simulink model "variant_2_MRC_SimulationModel"  (R2015a)
settings: Solver=ode3  SolverMode=SingleTasking  StartTime=0.0  StopTime=180  RelTol=1e-3
PreLoadFcn:
  | addLibrariesInPath('sim')
PostLoadFcn:
  | loadRobotParameters
StartFcn:
  | simApp = SimDisplay.getInstance;
  | simApp.reset;
  | simApp.TrackView.setup(double(SitesPositions), ObstaclesPositions,ObstaclesVertices,ObstaclesEdges);
undefined symbols (not defined in the file): AngularSpeed, AxleLength, do_one_run, EncL_init, EncR_init, EncRes, lcam, motorDeadBand, motorL, motorR, motorX, ObstaclesEdges, ObstaclesVertices, pcam, SitesPositions, startPos, TauMotor, theta0, Ts, WheelRadius
libraries: simulink_extras x1, realtime_pacer_lib x1, simulink x1, cstblocks x1
(part 1 of 2)
CloseFcn:
  | delete(SimDisplay.getInstance());
settings Model: PauseTimes=14  CovSFcnEnable=off  ExtModeTrigDuration=2  Creator=gpacitti  LastModifiedBy=planger
settings OptimizationCC: BlockReduction=off  BooleanDataType=off
settings DebuggingCC: SaveWithParameterizedLinksMsg=none  SignalResolutionControl=TryResolveAllWithWarning  ParameterPrecisionLossMsg=none
settings HardwareCC: TargetUnknown=on

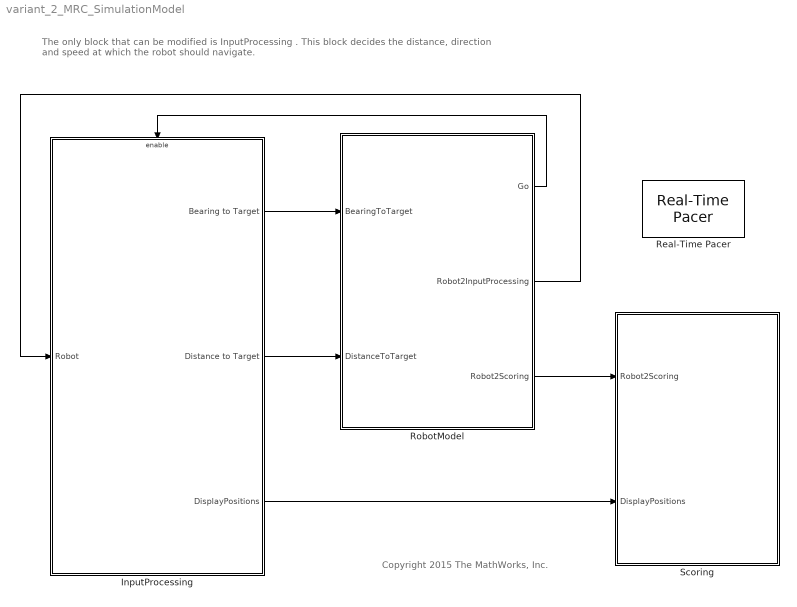
== system variant_2_MRC_SimulationModel ==
  note: Copyright 2015 The MathWorks, Inc.
  note: The only block that can be modified is InputProcessing .
      | This block decides the distance, direction and speed at which the robot should navigate.
  InputProcessing : Subsystem
      mask Display: image('Arduino_Due_2_0274.png',[0.15,0.3,0.45,0.4]);
  Real-Time Pacer : realtime_pacer_lib/Real-Time Pacer  simTimePerRealTime=1
  RobotModel : Subsystem  mask(Robot){}
      mask help:
      | !! DO NOT MODIFY !!
      | Model representing the robot behavior including physical representation and sensors.
      mask Display: image('robot_3d.jpg',[0.4,0.7,0.45,0.25]);
  Scoring : Subsystem  mask(Scoring){}
      mask help:
      | !! DO NOT MODIFY !!
      | Model representing the judge and visualisation.
  wires:
  InputProcessing/3(DisplayPositions) -> Scoring/2(DisplayPositions)
  InputProcessing/1(Bearing to Target) -> RobotModel/1(BearingToTarget)
  InputProcessing/2(Distance to Target) -> RobotModel/2(DistanceToTarget)
  RobotModel/2(Robot2InputProcessing) -> InputProcessing/1(Robot)
  RobotModel/3(Robot2Scoring) -> Scoring/1(Robot2Scoring)
  RobotModel/1(Go) -> InputProcessing/Enable

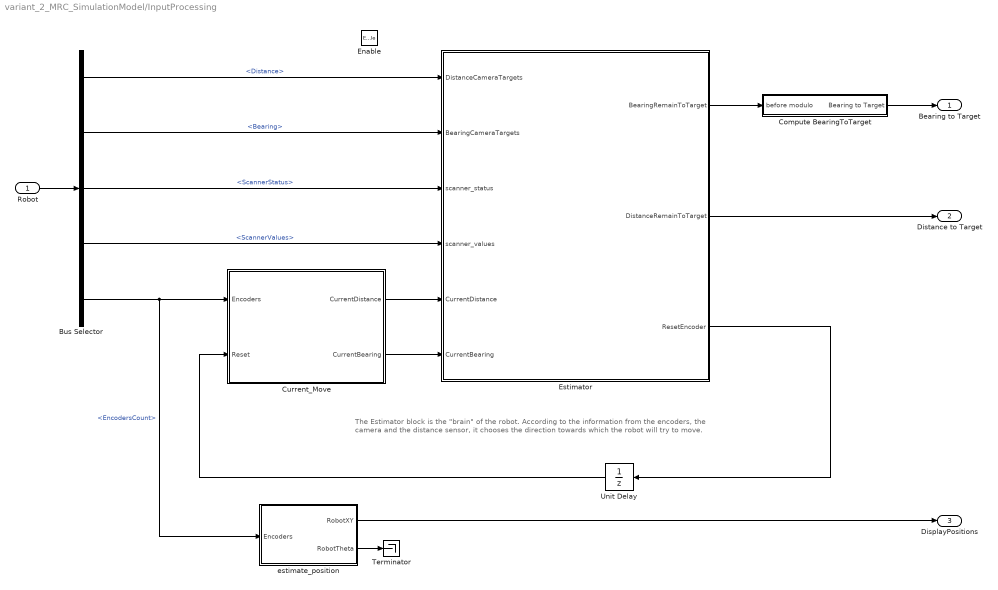
== system variant_2_MRC_SimulationModel/InputProcessing ==
  note: The Estimator block is the "brain" of the robot. According to the information from the encoders, the camera and the
      | distance sensor, it chooses the direction towards which the robot will try to move.
  Robot : Inport
  Enable : EnablePort  StatesWhenEnabling=reset
  Bus Selector : BusSelector  OutputSignals=Distance,Bearing,ScannerStatus,ScannerValues,EncodersCount
  Compute BearingToTarget : Subsystem
  Current_Move : Subsystem
  Estimator : Stateflow chart  TreatAsAtomicUnit=on
  Terminator : Terminator
  Unit Delay : UnitDelay  SampleTime=-1
  estimate_position : Subsystem
  Bearing to Target : Outport  SampleTime=Ts
  Distance to Target : Outport  Port=2
  DisplayPositions : Outport  Port=3
  wires:
  Robot/1 -> Bus Selector/1
  Bus Selector/1 -> Estimator/1(DistanceCameraTargets)  "<Distance>"
  Bus Selector/2 -> Estimator/2(BearingCameraTargets)  "<Bearing>"
  Estimator/1(BearingRemainToTarget) -> Compute BearingToTarget/1(before modulo)
  Estimator/2(DistanceRemainToTarget) -> Distance to Target/1
  Estimator/3(ResetEncoder) -> Unit Delay/1
  Unit Delay/1 -> Current_Move/2(Reset)
  Current_Move/1(CurrentDistance) -> Estimator/5(CurrentDistance)
  Compute BearingToTarget/1(Bearing to Target) -> Bearing to Target/1
  Current_Move/2(CurrentBearing) -> Estimator/6(CurrentBearing)
  estimate_position/2(RobotTheta) -> Terminator/1
  estimate_position/1(RobotXY) -> DisplayPositions/1
  Bus Selector/3 -> Estimator/3(scanner_status)  "<ScannerStatus>"
  Bus Selector/4 -> Estimator/4(scanner_values)  "<ScannerValues>"
  Bus Selector/5 -> estimate_position/1(Encoders), Current_Move/1(Encoders)  "<EncodersCount>"

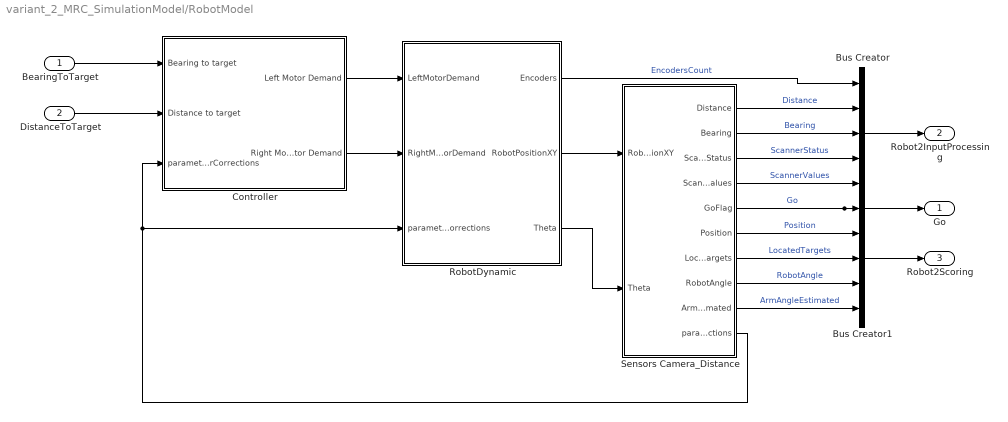
== system variant_2_MRC_SimulationModel/RobotModel ==
  BearingToTarget : Inport  SampleTime=0
  DistanceToTarget : Inport  Port=2  SampleTime=0
  Bus Creator : BusCreator  Inputs=5
  Bus Creator1 : BusCreator  Inputs=5
  Controller : Subsystem  TreatAsAtomicUnit=on
  RobotDynamic : Subsystem
  Sensors Camera_Distance : Subsystem
  Go : Outport
  Robot2InputProcessing : Outport  Port=2
  Robot2Scoring : Outport  Port=3
  wires:
  DistanceToTarget/1 -> Controller/2(Distance to target)
  BearingToTarget/1 -> Controller/1(Bearing to target)
  Bus Creator/1 -> Robot2InputProcessing/1
  Controller/1(Left Motor Demand) -> RobotDynamic/1(LeftMotorDemand)
  Controller/2(Right Motor Demand) -> RobotDynamic/2(RightMotorDemand)
  Bus Creator1/1 -> Robot2Scoring/1
  RobotDynamic/3(Theta) -> Sensors Camera_Distance/2(Theta)
  RobotDynamic/2(RobotPositionXY) -> Sensors Camera_Distance/1(RobotPositionXY)
  RobotDynamic/1(Encoders) -> Bus Creator/1  "EncodersCount"
  Sensors Camera_Distance/4(ScannerValues) -> Bus Creator/5  "ScannerValues"
  Sensors Camera_Distance/3(ScannerStatus) -> Bus Creator/4  "ScannerStatus"
  Sensors Camera_Distance/2(Bearing) -> Bus Creator/3  "Bearing"
  Sensors Camera_Distance/1(Distance) -> Bus Creator/2  "Distance"
  Sensors Camera_Distance/7(LocatedTargets) -> Bus Creator1/3  "LocatedTargets"
  Sensors Camera_Distance/8(RobotAngle) -> Bus Creator1/4  "RobotAngle"
  Sensors Camera_Distance/9(ArmAngleEstimated) -> Bus Creator1/5  "ArmAngleEstimated"
  Sensors Camera_Distance/10(parameterCorrections) -> RobotDynamic/3(parameterCorrections), Controller/3(parameterCorrections)
  Sensors Camera_Distance/6(Position) -> Bus Creator1/2  "Position"
  Sensors Camera_Distance/5(GoFlag) -> Bus Creator1/1, Go/1  "Go"

== system variant_2_MRC_SimulationModel/Scoring ==
  Robot2Scoring : Inport
  DisplayPositions : Inport  Port=2
  Bus Selector : BusSelector  OutputSignals=Position,Go
  Bus Selector1 : BusSelector  OutputSignals=LocatedTargets,RobotAngle,ArmAngleEstimated
  FigureOutput : Subsystem  TreatAsAtomicUnit=on  SimViewingDevice=on
  Referee : Subsystem
      mask Display: % image(imread('referee.png'))
  wires:
  Referee/1(Targets Located) -> FigureOutput/2(Targets Found)  "TargetsLocated"
  Referee/2(Time Last Target Found) -> FigureOutput/3(Time Last Found)  "TimeLastTargetFound"
  Referee/3(Elapsed Time_sec) -> FigureOutput/4(Time Elapsed)  "ElapsedTime"
  DisplayPositions/1 -> FigureOutput/9(DisplayPositions)
  Robot2Scoring/1 -> Bus Selector1/1, Bus Selector/1
  Bus Selector/2 -> Referee/2(Start Flag)  "<Go>"
  Bus Selector/1 -> FigureOutput/1(Position), Referee/1(Robot Position_m)  "<Position>"
  Bus Selector1/1 -> FigureOutput/5(locatedTargets)  "<LocatedTargets>"
  Bus Selector1/2 -> FigureOutput/6(robottheta)  "<RobotAngle>"
  Bus Selector1/3 -> FigureOutput/8(ArmAngleCommand), FigureOutput/7(ArmAngleEstimated)  "<ArmAngleEstimated>"

== system variant_2_MRC_SimulationModel/InputProcessing/Compute BearingToTarget ==
  before modulo : Inport
  Constant : Constant  Value=180  OutDataTypeStr=Inherit: Inherit via back propagation
  Constant1 : Constant  Value=360  OutDataTypeStr=Inherit: Inherit via back propagation
  Math Function1 : Math  Operator=mod  SaturateOnIntegerOverflow=on
  Sum10 : Sum  Inputs=-+|
  Sum7 : Sum  Inputs=++|
  Bearing to Target : Outport  SampleTime=Ts
  wires:
  Constant/1 -> Sum7/1, Sum10/1
  Sum7/1 -> Math Function1/1
  Constant1/1 -> Math Function1/2
  Math Function1/1 -> Sum10/2
  Sum10/1 -> Bearing to Target/1
  before modulo/1 -> Sum7/2

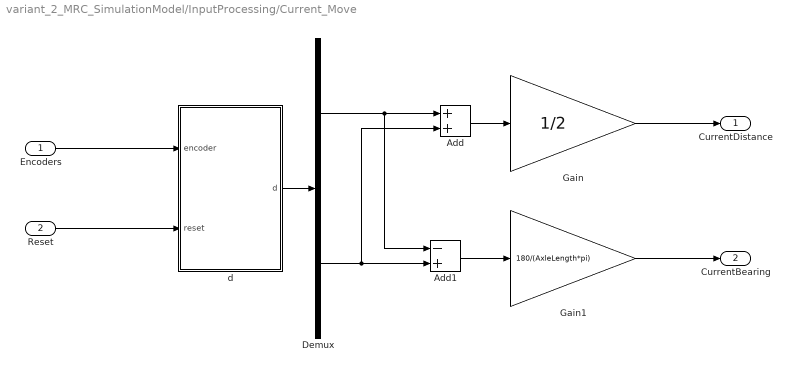
== system variant_2_MRC_SimulationModel/InputProcessing/Current_Move ==
  Encoders : Inport
  Reset : Inport  Port=2
  Add : Sum
  Add1 : Sum  Inputs=-+
  Demux : Demux  Outputs=2
  Gain : Gain  Gain=1/2
  Gain1 : Gain  Gain=180/(AxleLength*pi)
  d : Subsystem
  CurrentDistance : Outport
  CurrentBearing : Outport  Port=2
  wires:
  Reset/1 -> d/2(reset)
  Demux/2 -> Add/2, Add1/2
  Add1/1 -> Gain1/1
  Gain1/1 -> CurrentBearing/1
  Gain/1 -> CurrentDistance/1
  Demux/1 -> Add1/1, Add/1
  Add/1 -> Gain/1
  Encoders/1 -> d/1(encoder)
  d/1(d) -> Demux/1

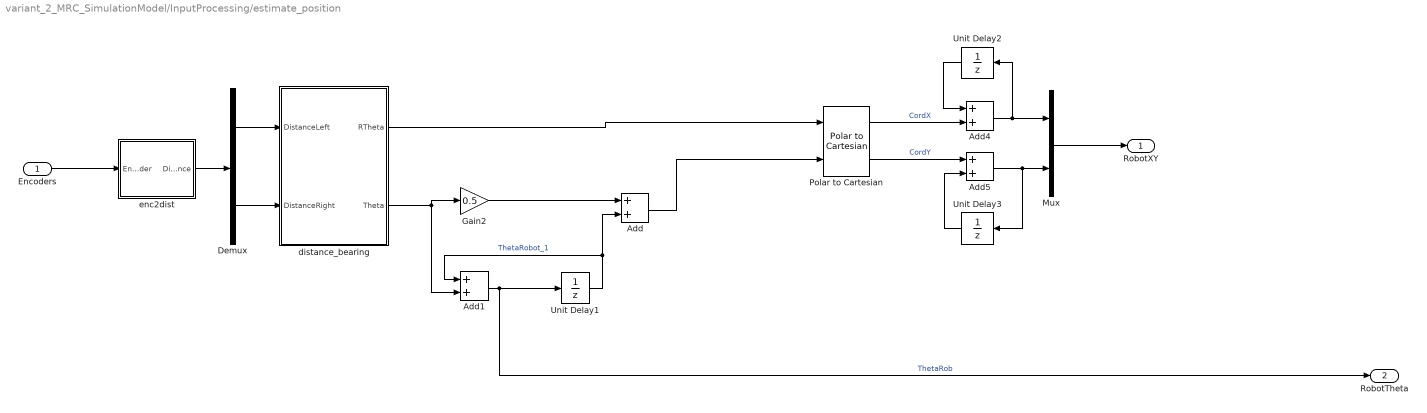
== system variant_2_MRC_SimulationModel/InputProcessing/estimate_position ==
  Encoders : Inport
  Add{,1,4..5} (4 alike) : Sum
  Demux : Demux  Outputs=2
  Gain2 : Gain  Gain=0.5
  Mux : Mux  Inputs=2
  Polar to Cartesian : simulink_extras/Transformations/Polar to Cartesian
  Unit Delay1 : UnitDelay  DialogController=Simulink.DDGSource  InitialCondition=theta0*pi/180  SampleTime=-1
  Unit Delay2 : UnitDelay  DialogController=Simulink.DDGSource  InitialCondition=single(startPos(1))  SampleTime=-1
  Unit Delay3 : UnitDelay  DialogController=Simulink.DDGSource  InitialCondition=single(startPos(2))  SampleTime=-1
  distance_bearing : Subsystem
  enc2dist : Subsystem
  RobotXY : Outport
  RobotTheta : Outport  Port=2
  wires:
  Gain2/1 -> Add/1
  Polar to Cartesian/1 -> Add4/2  "CordX"
  Polar to Cartesian/2 -> Add5/1  "CordY"
  Add4/1 -> Unit Delay2/1, Mux/1
  Unit Delay2/1 -> Add4/1
  Add5/1 -> Mux/2, Unit Delay3/1
  Unit Delay3/1 -> Add5/2
  distance_bearing/2(Theta) -> Gain2/1, Add1/2
  Unit Delay1/1 -> Add1/1, Add/2  "ThetaRobot_1"
  Add/1 -> Polar to Cartesian/2
  Add1/1 -> RobotTheta/1, Unit Delay1/1  "ThetaRob"
  distance_bearing/1(RTheta) -> Polar to Cartesian/1
  Mux/1 -> RobotXY/1
  enc2dist/1(Distance) -> Demux/1
  Demux/1 -> distance_bearing/1(DistanceLeft)
  Demux/2 -> distance_bearing/2(DistanceRight)
  Encoders/1 -> enc2dist/1(Encoder)

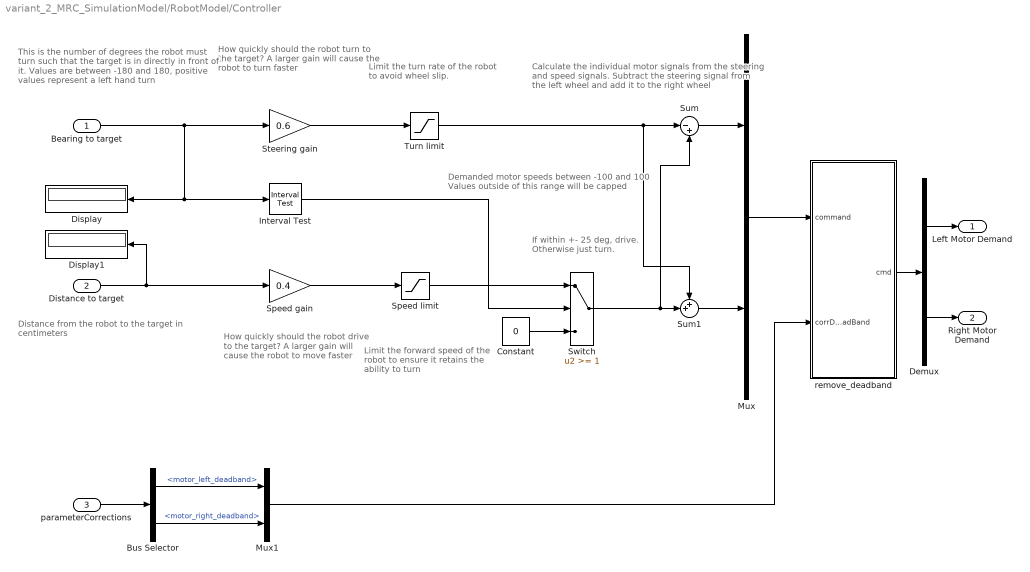
== system variant_2_MRC_SimulationModel/RobotModel/Controller ==
  note: Limit the turn rate of the
      | robot to avoid wheel slip.
  note: If within +- 25 deg, drive.
      | Otherwise just turn.
  note: Calculate the individual motor signals from the
      | steering and speed signals. Subtract the steering
      | signal from the left wheel and add it to the right
      | wheel
  note: Limit the forward speed of the
      | robot to ensure it retains the
      | ability to turn
  note: How quickly should the robot
      | drive to the target? A larger gain
      | will cause the robot to move
      | faster
  note: How quickly should the robot turn
      | to the target? A larger gain will
      |  cause the robot to turn faster
  note: Demanded motor speeds between -100 and 100
      | Values outside of this range will be capped
  note: Distance from the robot to the target
      | in centimeters
  note: This is the number of degrees the robot
      | must turn such that the target is in directly
      | in front of it.
      | Values are between -180 and 180,
      | positive values represent a left hand turn
  Bearing to target : Inport  OutDataTypeStr=single
  Distance to target : Inport  Port=2  PortDimensions=1  SampleTime=Ts
  parameterCorrections : Inport  Port=3  SampleTime=Ts
  Bus Selector : BusSelector  OutputSignals=motor_left_deadband,motor_right_deadband
  Constant : Constant  Value=0  OutDataTypeStr=single
  Demux : Demux  Outputs=2
  Display : Display
  Display1 : Display
  Interval Test : simulink/Logic and Bit Operations/Interval Test  IntervalClosedRight=on  uplimit=25  IntervalClosedLeft=on  lowlimit=-25  OutDataTypeStr=boolean
      settings: AttributesFormatString=|
      | Upper = %<uplimit>
      | Lower = %<lowlimit>
  Mux : Mux  Inputs=2
  Mux1 : Mux  Inputs=2
  Speed gain : Gain  Gain=0.4
  Speed limit : Saturate  UpperLimit=40  LowerLimit=0
      settings: AttributesFormatString=|
      | Upper = %<UpperLimit>
      | Lower = %<LowerLimit>
  Steering gain : Gain  Gain=0.6
  Sum : Sum  Inputs=|-+
  Sum1 : Sum  Inputs=++|
  Switch : Switch  Threshold=1
  Turn limit : Saturate  UpperLimit=50  LowerLimit=-50
      settings: AttributesFormatString=|
      | Upper = %<UpperLimit>
      | Lower = %<LowerLimit>
  remove_deadband : Subsystem
  Left Motor Demand : Outport  OutDataTypeStr=single
  Right Motor Demand : Outport  Port=2  OutDataTypeStr=single
  wires:
  Bearing to target/1 -> Steering gain/1, Display/1, Interval Test/1
  Speed gain/1 -> Speed limit/1
  Distance to target/1 -> Display1/1, Speed gain/1
  Steering gain/1 -> Turn limit/1
  Switch/1 -> Sum/2, Sum1/2
  Interval Test/1 -> Switch/2
  Constant/1 -> Switch/3
  Turn limit/1 -> Sum/1, Sum1/1
  Speed limit/1 -> Switch/1
  parameterCorrections/1 -> Bus Selector/1
  Sum1/1 -> Mux/2
  Sum/1 -> Mux/1
  Mux/1 -> remove_deadband/1(command)
  remove_deadband/1(cmd) -> Demux/1
  Demux/1 -> Left Motor Demand/1
  Demux/2 -> Right Motor Demand/1
  Bus Selector/1 -> Mux1/1  "<motor_left_deadband>"
  Bus Selector/2 -> Mux1/2  "<motor_right_deadband>"
  Mux1/1 -> remove_deadband/2(corrDeadBand)

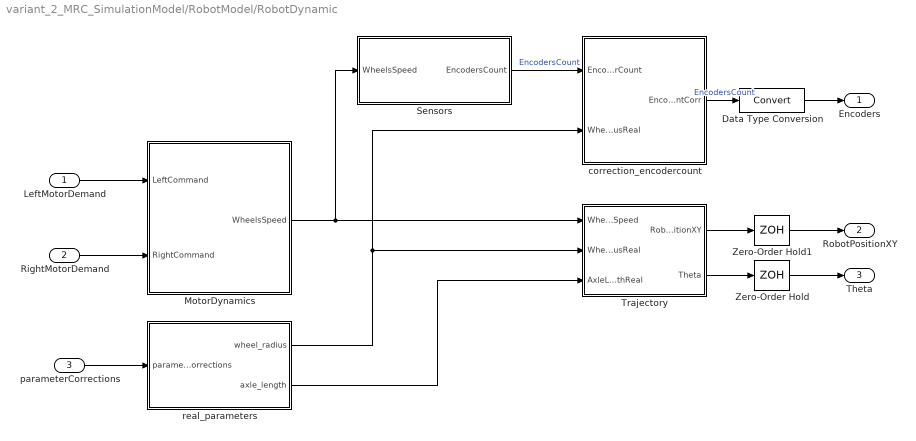
== system variant_2_MRC_SimulationModel/RobotModel/RobotDynamic ==
  LeftMotorDemand : Inport
  RightMotorDemand : Inport  Port=2
  parameterCorrections : Inport  Port=3
  Data Type Conversion : DataTypeConversion
  MotorDynamics : Subsystem
  Sensors : Subsystem
  Trajectory : Subsystem
  Zero-Order Hold : ZeroOrderHold  SampleTime=Ts
  Zero-Order Hold1 : ZeroOrderHold  SampleTime=Ts
  correction_encodercount : Subsystem
  real_parameters : Subsystem
  Encoders : Outport
  RobotPositionXY : Outport  Port=2
  Theta : Outport  Port=3
  wires:
  MotorDynamics/1(WheelsSpeed) -> Trajectory/1(WheelsSpeed), Sensors/1(WheelsSpeed)
  RightMotorDemand/1 -> MotorDynamics/2(RightCommand)
  LeftMotorDemand/1 -> MotorDynamics/1(LeftCommand)
  correction_encodercount/1(EncoderCountCorr) -> Data Type Conversion/1  "EncodersCount"
  Trajectory/1(RobotPositionXY) -> Zero-Order Hold1/1
  Trajectory/2(Theta) -> Zero-Order Hold/1
  Zero-Order Hold1/1 -> RobotPositionXY/1
  Zero-Order Hold/1 -> Theta/1
  parameterCorrections/1 -> real_parameters/1(parameterCorrections)
  Sensors/1(EncodersCount) -> correction_encodercount/1(EncoderCount)  "EncodersCount"
  real_parameters/2(axle_length) -> Trajectory/3(AxleLengthReal)
  real_parameters/1(wheel_radius) -> Trajectory/2(WheelsRadiusReal), correction_encodercount/2(WheelRadiusReal)
  Data Type Conversion/1 -> Encoders/1

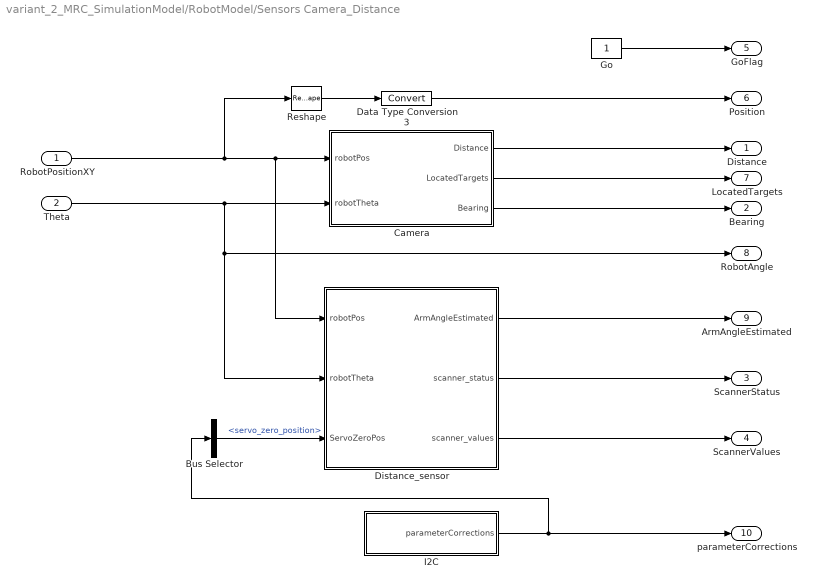
== system variant_2_MRC_SimulationModel/RobotModel/Sensors Camera_Distance ==
  RobotPositionXY : Inport
  Theta : Inport  Port=2
  Bus Selector : BusSelector  OutputSignals=servo_zero_position
  Camera : Subsystem
  Data Type Conversion3 : DataTypeConversion
  Distance_sensor : Subsystem
  Go : Constant  OutMin=0  OutMax=1  OutDataTypeStr=boolean  SampleTime=0.1
  I2C : Subsystem
  Reshape : Reshape  OutputDimensionality=Row vector (2-D)
  Distance : Outport  OutDataTypeStr=int16
  Bearing : Outport  Port=2  OutDataTypeStr=int8
  ScannerStatus : Outport  Port=3
  ScannerValues : Outport  Port=4
  GoFlag : Outport  Port=5
  Position : Outport  Port=6
  LocatedTargets : Outport  Port=7
  RobotAngle : Outport  Port=8
  ArmAngleEstimated : Outport  Port=9
  parameterCorrections : Outport  Port=10
  wires:
  Data Type Conversion3/1 -> Position/1
  Reshape/1 -> Data Type Conversion3/1
  RobotPositionXY/1 -> Distance_sensor/1(robotPos), Camera/1(robotPos), Reshape/1
  Theta/1 -> RobotAngle/1, Distance_sensor/2(robotTheta), Camera/2(robotTheta)
  Camera/1(Distance) -> Distance/1
  Camera/2(LocatedTargets) -> LocatedTargets/1
  Camera/3(Bearing) -> Bearing/1
  Distance_sensor/1(ArmAngleEstimated) -> ArmAngleEstimated/1
  Distance_sensor/2(scanner_status) -> ScannerStatus/1
  Distance_sensor/3(scanner_values) -> ScannerValues/1
  I2C/1(parameterCorrections) -> Bus Selector/1, parameterCorrections/1
  Bus Selector/1 -> Distance_sensor/3(ServoZeroPos)  "<servo_zero_position>"
  Go/1 -> GoFlag/1

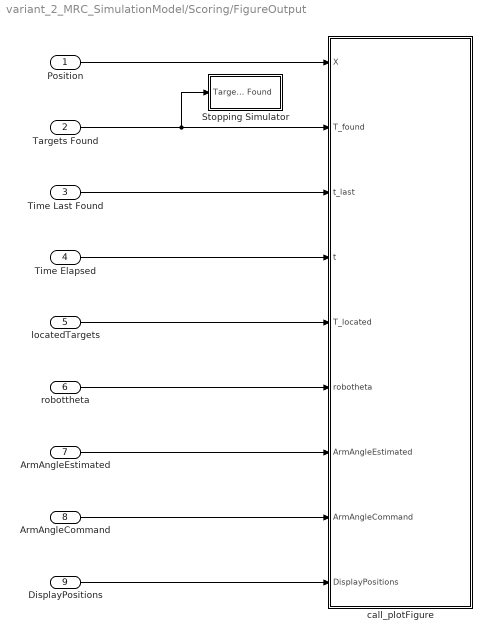
== system variant_2_MRC_SimulationModel/Scoring/FigureOutput ==
  Position : Inport
  Targets Found : Inport  Port=2
  Time Last Found : Inport  Port=3
  Time Elapsed : Inport  Port=4
  locatedTargets : Inport  Port=5
  robottheta : Inport  Port=6
  ArmAngleEstimated : Inport  Port=7
  ArmAngleCommand : Inport  Port=8
  DisplayPositions : Inport  Port=9
  Stopping Simulator : Subsystem
  call_plotFigure : MATLAB Function  TreatAsAtomicUnit=on
  wires:
  Position/1 -> call_plotFigure/1(X)
  Targets Found/1 -> Stopping Simulator/1(Targets Found), call_plotFigure/2(T_found)
  Time Last Found/1 -> call_plotFigure/3(t_last)
  Time Elapsed/1 -> call_plotFigure/4(t)
  locatedTargets/1 -> call_plotFigure/5(T_located)
  robottheta/1 -> call_plotFigure/6(robotheta)
  DisplayPositions/1 -> call_plotFigure/9(DisplayPositions)
  ArmAngleEstimated/1 -> call_plotFigure/7(ArmAngleEstimated)
  ArmAngleCommand/1 -> call_plotFigure/8(ArmAngleCommand)

== system variant_2_MRC_SimulationModel/Scoring/Referee ==
  Robot Position_m : Inport  SampleTime=Ts
  Start Flag : Inport  Port=2  OutDataTypeStr=boolean  SampleTime=Ts
  Digital Clock1 : DigitalClock  SampleTime=Ts
  Referee : Stateflow chart  TreatAsAtomicUnit=on
  Reshape : Reshape  OutputDimensionality=Row vector (2-D)
  Targets Located : Outport
  Time Last Target Found : Outport  Port=2  PortDimensions=1
  Elapsed Time_sec : Outport  Port=3  PortDimensions=1
  wires:
  Referee/1(timeLastTargetFound) -> Time Last Target Found/1
  Referee/3(targetsFound) -> Targets Located/1
  Robot Position_m/1 -> Reshape/1
  Start Flag/1 -> Referee/2(StartFlag)
  Reshape/1 -> Referee/1(robotPosition)
  Referee/2(elapsedTime) -> Elapsed Time_sec/1
  Digital Clock1/1 -> Referee/3(sim_time)

== system variant_2_MRC_SimulationModel/InputProcessing/Current_Move/d ==
  encoder : Inport
  reset : Inport  Port=2
  Add : Sum  Inputs=-+  OutDataTypeStr=single
  Gain : Gain  Gain=2*pi/EncRes
  Product : Product
  Triggered Subsystem : Subsystem  TreatAsAtomicUnit=on
  WheelRadius : Constant  Value=WheelRadius  OutDataTypeStr=Inherit: Inherit via back propagation
  d : Outport
  wires:
  Triggered Subsystem/1(encoderTarget) -> Add/1
  reset/1 -> Triggered Subsystem/Trigger
  encoder/1 -> Triggered Subsystem/1(encoderIn), Add/2
  Gain/1 -> d/1
  Add/1 -> Product/2
  Product/1 -> Gain/1
  WheelRadius/1 -> Product/1

== system variant_2_MRC_SimulationModel/InputProcessing/estimate_position/distance_bearing ==
  DistanceLeft : Inport
  DistanceRight : Inport  Port=2
  Add : Sum
  Add1 : Sum  Inputs=-+
  Gain : Gain  Gain=0.5
  Gain1 : Gain  Gain=1/AxleLength
  RTheta : Outport
  Theta : Outport  Port=2
  wires:
  Gain1/1 -> Theta/1
  Add/1 -> Gain/1
  Gain/1 -> RTheta/1
  Add1/1 -> Gain1/1
  DistanceLeft/1 -> Add1/1, Add/1
  DistanceRight/1 -> Add/2, Add1/2

== system variant_2_MRC_SimulationModel/InputProcessing/estimate_position/enc2dist ==
  Encoder : Inport
  Add2 : Sum  Inputs=-+
  Gain : Gain  Gain=2*pi/EncRes  OutDataTypeStr=single
  Product : Product
  Unit Delay : UnitDelay  DialogController=Simulink.DDGSource  SampleTime=-1
  WheelRadius : Constant  Value=WheelRadius  OutDataTypeStr=single
  Distance : Outport
  wires:
  Product/1 -> Gain/1
  Encoder/1 -> Product/1
  Gain/1 -> Unit Delay/1, Add2/2
  Unit Delay/1 -> Add2/1
  Add2/1 -> Distance/1
  WheelRadius/1 -> Product/2

== system variant_2_MRC_SimulationModel/RobotModel/Controller/remove_deadband ==
  command : Inport
  corrDeadBand : Inport  Port=2
  Add : Sum
  Add1 : Sum
  Product : Product
  Sign : Signum
  motorDeadBand : Constant  Value=motorDeadBand  OutDataTypeStr=Inherit: Inherit via back propagation
  cmd : Outport
  wires:
  Product/1 -> Add/2
  Add/1 -> cmd/1
  Sign/1 -> Product/1
  command/1 -> Sign/1, Add/1
  motorDeadBand/1 -> Add1/1
  corrDeadBand/1 -> Add1/2
  Add1/1 -> Product/2

== system variant_2_MRC_SimulationModel/RobotModel/RobotDynamic/MotorDynamics ==
  LeftCommand : Inport
  RightCommand : Inport  Port=2
  Dynamics : cstblocks/LTI System  sys=tf(1,[TauMotor 1])*eye(2)  IC=[]
  Left_motor_table : Lookup_n-D  NumberOfTableDimensions=1  BreakpointsForDimension1=motorX  Table=motorL  ExtrapMethod=Clip  InternalRulePriority=Speed  OutDataTypeStr=Inherit: Inherit via back propagation  RndMeth=Simplest  InputSameDT=on
  Mux1 : Mux  Inputs=2
  Right_motor_table : Lookup_n-D  NumberOfTableDimensions=1  BreakpointsForDimension1=motorX  Table=motorR  ExtrapMethod=Clip  InternalRulePriority=Speed  OutDataTypeStr=Inherit: Inherit via back propagation  RndMeth=Simplest  InputSameDT=on
  WheelsSpeed : Outport  PortDimensions=2
  wires:
  Dynamics/1 -> WheelsSpeed/1  "Wheels Velocity d°/s"
  LeftCommand/1 -> Left_motor_table/1
  RightCommand/1 -> Right_motor_table/1
  Right_motor_table/1 -> Mux1/2
  Left_motor_table/1 -> Mux1/1
  Mux1/1 -> Dynamics/1  "Speed Demand d°/s"

== system variant_2_MRC_SimulationModel/RobotModel/RobotDynamic/Sensors ==
  WheelsSpeed : Inport
  Encoder Quantization : Quantizer  QuantizationInterval=(360/EncRes)
  Encoder Reading : ZeroOrderHold  SampleTime=Ts
  angular_position : Integrator  InitialCondition=[EncL_init;EncR_init]
  deg2encoderCount : Gain  Gain=EncRes/360  OutDataTypeStr=Inherit: Inherit via back propagation
  EncodersCount : Outport
  wires:
  WheelsSpeed/1 -> angular_position/1  "Wheels Velocity d°/s"
  Encoder Reading/1 -> Encoder Quantization/1
  angular_position/1 -> deg2encoderCount/1  "WheelsPosition d°"
  Encoder Quantization/1 -> EncodersCount/1
  deg2encoderCount/1 -> Encoder Reading/1

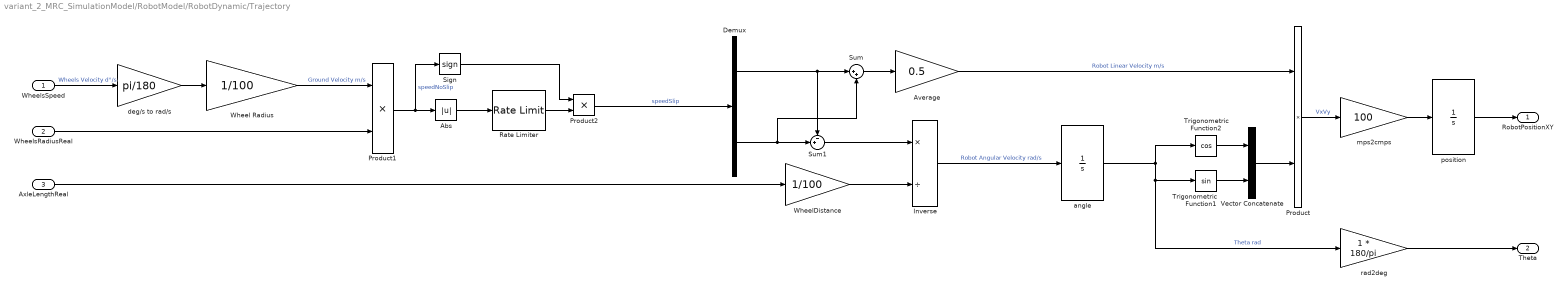
== system variant_2_MRC_SimulationModel/RobotModel/RobotDynamic/Trajectory ==
  WheelsSpeed : Inport  PortDimensions=2
  WheelsRadiusReal : Inport  Port=2  PortDimensions=2
  AxleLengthReal : Inport  Port=3  PortDimensions=1
  Abs : Abs
  Average : Gain  Gain=0.5
  Demux : Demux  Outputs=2
  Inverse : Product  Inputs=*/
  Product : Product
  Product1 : Product
  Product2 : Product
  Rate Limiter : RateLimiter  RisingSlewLimit=[1 1.2]  FallingSlewLimit=-1000  SampleTimeMode=inherited
  Sign : Signum
  Sum : Sum  Inputs=|++
  Sum1 : Sum  Inputs=-+|
  Trigonometric Function1 : Trigonometry
  Trigonometric Function2 : Trigonometry  Operator=cos
  Vector Concatenate : Concatenate
  Wheel Radius : Gain  Gain=1/100
  WheelDistance : Gain  Gain=1/100
  angle : Integrator  InitialCondition=theta0 * pi/180
  deg/s to rad/s : Gain  Gain=pi/180
  mps2cmps : Gain  Gain=100
  position : Integrator  InitialCondition=double(startPos)
  rad2deg : Gain  Gain=1 * 180/pi
  RobotPositionXY : Outport
  Theta : Outport  Port=2
  wires:
  angle/1 -> rad2deg/1, Trigonometric Function1/1, Trigonometric Function2/1  "Theta rad"
  Trigonometric Function2/1 -> Vector Concatenate/1
  Trigonometric Function1/1 -> Vector Concatenate/2
  Vector Concatenate/1 -> Product/2
  Average/1 -> Product/1  "Robot Linear Velocity m/s"
  Sum/1 -> Average/1
  Demux/2 -> Sum1/2, Sum/2
  Demux/1 -> Sum1/1, Sum/1
  Sum1/1 -> Inverse/1
  Product/1 -> mps2cmps/1  "VxVy"
  Inverse/1 -> angle/1  "Robot Angular Velocity rad/s"
  deg/s to rad/s/1 -> Wheel Radius/1
  mps2cmps/1 -> position/1
  position/1 -> RobotPositionXY/1
  rad2deg/1 -> Theta/1
  WheelsSpeed/1 -> deg/s to rad/s/1  "Wheels Velocity d°/s"
  AxleLengthReal/1 -> WheelDistance/1
  Wheel Radius/1 -> Product1/1  "Ground Velocity m/s"
  WheelsRadiusReal/1 -> Product1/2
  WheelDistance/1 -> Inverse/2
  Product1/1 -> Sign/1, Abs/1  "speedNoSlip"
  Product2/1 -> Demux/1  "speedSlip"
  Abs/1 -> Rate Limiter/1
  Rate Limiter/1 -> Product2/2
  Sign/1 -> Product2/1

== system variant_2_MRC_SimulationModel/RobotModel/RobotDynamic/correction_encodercount ==
  EncoderCount : Inport
  WheelRadiusReal : Inport  Port=2
  Divide : Product  Inputs=*/
  Product : Product
  WheelRadius : Constant  Value=WheelRadius
  EncoderCountCorr : Outport
  wires:
  WheelRadius/1 -> Divide/1  "wheelRadius_ideal"
  Divide/1 -> Product/2  "corr_factor"
  EncoderCount/1 -> Product/1  "measured"
  Product/1 -> EncoderCountCorr/1  "corrected"
  WheelRadiusReal/1 -> Divide/2

== system variant_2_MRC_SimulationModel/RobotModel/RobotDynamic/real_parameters ==
  parameterCorrections : Inport
  Add : Sum
  Add1 : Sum
  AxleLength : Constant  Value=AxleLength
  Bus Selector : BusSelector  OutputSignals=wheel_left_diameter,wheel_right_diameter
  Bus Selector1 : BusSelector  OutputSignals=axle_length
  Mux : Mux  Inputs=2
  WheelRadius : Constant  Value=WheelRadius
  wheel_radius : Outport
  axle_length : Outport  Port=2
  wires:
  Add/1 -> wheel_radius/1
  WheelRadius/1 -> Add/1
  parameterCorrections/1 -> Bus Selector1/1, Bus Selector/1
  Bus Selector/1 -> Mux/1  "<wheel_left_diameter>"
  Bus Selector/2 -> Mux/2  "<wheel_right_diameter>"
  Mux/1 -> Add/2
  Bus Selector1/1 -> Add1/2  "<axle_length>"
  AxleLength/1 -> Add1/1
  Add1/1 -> axle_length/1

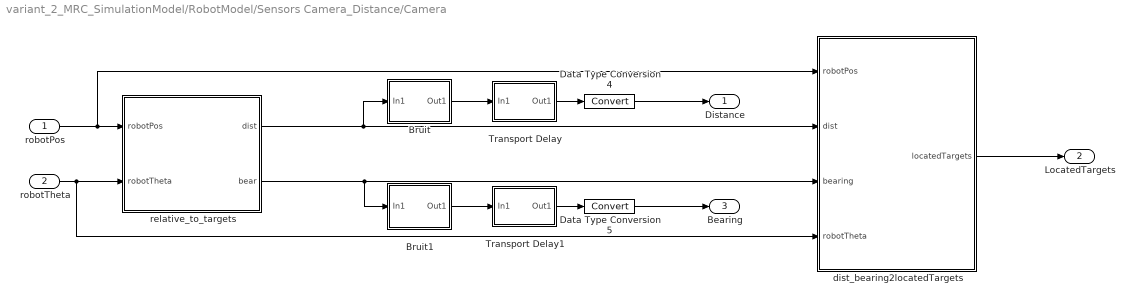
== system variant_2_MRC_SimulationModel/RobotModel/Sensors Camera_Distance/Camera ==
  robotPos : Inport
  robotTheta : Inport  Port=2
  Bruit : Subsystem
  Bruit1 : Subsystem
  Data Type Conversion4 : DataTypeConversion
  Data Type Conversion5 : DataTypeConversion
  Transport Delay : Subsystem  mask{timeDelay=0.300, initialOutput=zeros(size(6,1),1), initialBufferSize=1024, useFixedBufferSize=off, directFeedthoughOfInputDuringLinearization=off, padeOrder=0}
      mask prompts: initialOutput "Initial output"; initialBufferSize "Initial buffer size"; useFixedBufferSize "Use fixed buffer size"; directFeedthoughOfInputDuringLinearization "Direct feedthough of input during linearization"; padeOrder "Pade order (for linearization):"
  Transport Delay1 : Subsystem  mask{timeDelay=0.300, initialOutput=zeros(size(6,1),1), initialBufferSize=1024, useFixedBufferSize=off, directFeedthoughOfInputDuringLinearization=off, padeOrder=0}
      mask prompts: initialOutput "Initial output"; initialBufferSize "Initial buffer size"; useFixedBufferSize "Use fixed buffer size"; directFeedthoughOfInputDuringLinearization "Direct feedthough of input during linearization"; padeOrder "Pade order (for linearization):"
  dist_bearing2locatedTargets : MATLAB Function  TreatAsAtomicUnit=on
  relative_to_targets : MATLAB Function  TreatAsAtomicUnit=on
  Distance : Outport  OutDataTypeStr=int16
  LocatedTargets : Outport  Port=2
  Bearing : Outport  Port=3  OutDataTypeStr=int8
  wires:
  Transport Delay/1(Out1) -> Data Type Conversion4/1
  Data Type Conversion4/1 -> Distance/1
  relative_to_targets/2(bear) -> Bruit1/1(In1), dist_bearing2locatedTargets/3(bearing)
  dist_bearing2locatedTargets/1(locatedTargets) -> LocatedTargets/1
  Transport Delay1/1(Out1) -> Data Type Conversion5/1
  Bruit1/1(Out1) -> Transport Delay1/1(In1)
  relative_to_targets/1(dist) -> Bruit/1(In1), dist_bearing2locatedTargets/2(dist)
  Bruit/1(Out1) -> Transport Delay/1(In1)
  Data Type Conversion5/1 -> Bearing/1
  robotTheta/1 -> dist_bearing2locatedTargets/4(robotTheta), relative_to_targets/2(robotTheta)
  robotPos/1 -> dist_bearing2locatedTargets/1(robotPos), relative_to_targets/1(robotPos)

== system variant_2_MRC_SimulationModel/RobotModel/Sensors Camera_Distance/Distance_sensor ==
  robotPos : Inport  SampleTime=Ts
  robotTheta : Inport  Port=2  SampleTime=Ts
  ServoZeroPos : Inport  Port=3  SampleTime=Ts
  ArmAngleEstimator : Subsystem
  Scanner : Stateflow chart  TreatAsAtomicUnit=on
  arm_distance : MATLAB Function  TreatAsAtomicUnit=on
  ArmAngleEstimated : Outport
  scanner_status : Outport  Port=2
  scanner_values : Outport  Port=3
  wires:
  ServoZeroPos/1 -> ArmAngleEstimator/1("  ServoZeroPos")
  ArmAngleEstimator/1(ArmAngleEstimated) -> arm_distance/3(armAngle), ArmAngleEstimated/1
  robotTheta/1 -> arm_distance/2(robotTheta)
  robotPos/1 -> arm_distance/1(robotPos)
  Scanner/3(ArmAngle) -> ArmAngleEstimator/2("  ArmAngleCommand")
  arm_distance/1(armDist) -> Scanner/1(ArmDist)
  Scanner/2(scanner_value) -> scanner_values/1
  Scanner/1(scanner_status) -> scanner_status/1

== system variant_2_MRC_SimulationModel/RobotModel/Sensors Camera_Distance/I2C ==
  Bus Creator : BusCreator  Inputs=6
  axle_length : Constant  Value=0  OutDataTypeStr=Inherit: Inherit via back propagation
  motor_left_deadband : Constant  Value=0  OutDataTypeStr=Inherit: Inherit via back propagation
  motor_right_deadband : Constant  Value=0  OutDataTypeStr=Inherit: Inherit via back propagation
  servo_zero_position : Constant  Value=0  OutDataTypeStr=Inherit: Inherit via back propagation
  wheel_left_diameter : Constant  Value=0  OutDataTypeStr=Inherit: Inherit via back propagation
  wheel_right_diameter : Constant  Value=0  OutDataTypeStr=Inherit: Inherit via back propagation
  parameterCorrections : Outport
  wires:
  wheel_left_diameter/1 -> Bus Creator/1  "wheel_left_diameter"
  Bus Creator/1 -> parameterCorrections/1
  motor_right_deadband/1 -> Bus Creator/4  "motor_right_deadband"
  motor_left_deadband/1 -> Bus Creator/3  "motor_left_deadband"
  wheel_right_diameter/1 -> Bus Creator/2  "wheel_right_diameter"
  servo_zero_position/1 -> Bus Creator/5  "servo_zero_position"
  axle_length/1 -> Bus Creator/6  "axle_length"

== system variant_2_MRC_SimulationModel/Scoring/FigureOutput/Stopping Simulator ==
  Targets Found : Inport
  Constant : Constant  Value=do_one_run
  Data Type Conversion : DataTypeConversion  OutDataTypeStr=double
  Logical Operator1 : Logic  AllPortsSameDT=off  OutDataTypeStr=boolean
  MinMax : MinMax
  Stop Simulation : Stop
  wires:
  Targets Found/1 -> Data Type Conversion/1
  Data Type Conversion/1 -> MinMax/1
  MinMax/1 -> Logical Operator1/1
  Constant/1 -> Logical Operator1/2
  Logical Operator1/1 -> Stop Simulation/1

== system variant_2_MRC_SimulationModel/InputProcessing/Current_Move/d/Triggered Subsystem ==
  encoderIn : Inport
  Trigger : TriggerPort  TriggerType=either
  encoderTarget : Outport
  wires:
  encoderIn/1 -> encoderTarget/1

== system variant_2_MRC_SimulationModel/RobotModel/Sensors Camera_Distance/Camera/Bruit ==
  In1 : Inport
  Add : Sum
  Data Type Conversion4 : DataTypeConversion
  Product : Product
  Uniform Random Number : UniformRandomNumber  Minimum=-0.05  Maximum=0.05  SampleTime=Ts
  Out1 : Outport
  wires:
  In1/1 -> Add/2, Product/2
  Product/1 -> Add/1
  Uniform Random Number/1 -> Data Type Conversion4/1
  Data Type Conversion4/1 -> Product/1
  Add/1 -> Out1/1

== system variant_2_MRC_SimulationModel/RobotModel/Sensors Camera_Distance/Camera/Bruit1 ==
  In1 : Inport
  Add : Sum
  Data Type Conversion4 : DataTypeConversion
  Product : Product
  Uniform Random Number : UniformRandomNumber  Minimum=-0.05  Maximum=0.05  SampleTime=Ts
  Out1 : Outport
  wires:
  Data Type Conversion4/1 -> Product/1
  Uniform Random Number/1 -> Data Type Conversion4/1
  Product/1 -> Add/1
  In1/1 -> Add/2, Product/2
  Add/1 -> Out1/1

== system variant_2_MRC_SimulationModel/RobotModel/Sensors Camera_Distance/Camera/Transport Delay ==
  In1 : Inport
  Data Type Conversion : DataTypeConversion  OutDataTypeStr=double
  Data Type Conversion4 : DataTypeConversion  OutDataTypeStr=single
  Transport Delay : TransportDelay  DelayTime=timeDelay  InitialOutput=initialOutput  BufferSize=initialBufferSize  PadeOrder=padeOrder
  Zero-Order Hold : ZeroOrderHold  SampleTime=Ts
  Out1 : Outport
  wires:
  Transport Delay/1 -> Data Type Conversion4/1
  Data Type Conversion/1 -> Transport Delay/1
  Data Type Conversion4/1 -> Zero-Order Hold/1
  In1/1 -> Data Type Conversion/1
  Zero-Order Hold/1 -> Out1/1

== system variant_2_MRC_SimulationModel/RobotModel/Sensors Camera_Distance/Camera/Transport Delay1 ==
  In1 : Inport
  Data Type Conversion : DataTypeConversion  OutDataTypeStr=double
  Data Type Conversion4 : DataTypeConversion  OutDataTypeStr=single
  Transport Delay : TransportDelay  DelayTime=timeDelay  InitialOutput=initialOutput  BufferSize=initialBufferSize  PadeOrder=padeOrder
  Zero-Order Hold : ZeroOrderHold  SampleTime=Ts
  Out1 : Outport
  wires:
  In1/1 -> Data Type Conversion/1
  Data Type Conversion4/1 -> Zero-Order Hold/1
  Data Type Conversion/1 -> Transport Delay/1
  Transport Delay/1 -> Data Type Conversion4/1
  Zero-Order Hold/1 -> Out1/1

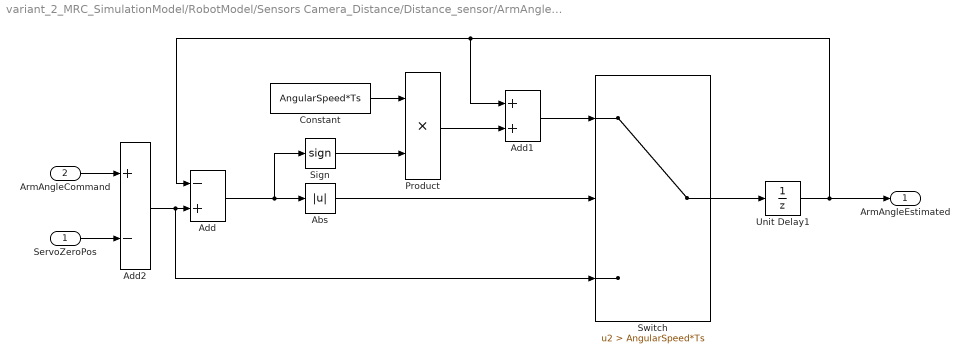
== system variant_2_MRC_SimulationModel/RobotModel/Sensors Camera_Distance/Distance_sensor/ArmAngleEstimator ==
  "  ServoZeroPos" : Inport
  "  ArmAngleCommand" : Inport  Port=2
  Abs : Abs
  Add : Sum  Inputs=-+
  Add1 : Sum
  Add2 : Sum  Inputs=+-
  Constant : Constant  Value=AngularSpeed*Ts
  Product : Product
  Sign : Signum
  Switch : Switch  Criteria=u2 > Threshold  Threshold=AngularSpeed*Ts
  Unit Delay1 : UnitDelay  DialogController=Simulink.DDGSource  SampleTime=-1
  ArmAngleEstimated : Outport
  wires:
  Add/1 -> Sign/1, Abs/1
  Abs/1 -> Switch/2
  Switch/1 -> Unit Delay1/1
  Constant/1 -> Product/1
  Sign/1 -> Product/2
  Product/1 -> Add1/2
  Add1/1 -> Switch/1
  Unit Delay1/1 -> Add/1, Add1/1, ArmAngleEstimated/1
  "  ServoZeroPos"/1 -> Add2/2
  Add2/1 -> Switch/3, Add/2
  "  ArmAngleCommand"/1 -> Add2/1

== matlab function variant_2_MRC_SimulationModel/RobotModel/Sensors Camera_Distance/Distance_sensor/arm_distance ==
  data: robotPos input size=[1 2]; robotTheta input size=1; armAngle input; ObstaclesVertices parameter; ObstaclesEdges parameter; armDist output
 function armDist  = targets(robotPos,robotTheta,armAngle,ObstaclesVertices, ObstaclesEdges)
%#codegen
%% TARGETS Returns distance and bearing for each target relative tos robot
%
% Distances and positions are in cm
% Angles are in degrees
%
% Inputs
%   - hCam: Cam height (from ground)
%   - targetsPos: Position of targets (X,Y)
%   - robotPos: Robot position (X,Y)
%   - robotTheta: Robot angle
%
% Outputs
%   - dist (array nx1 with n=nb targets): Distances for each target,
%       if a target cannot be seen by the camera associated distance
%       is equal to -1
%   - bearing (array nx1 with n=nb targets): Angles for each target,
%       if a target cannot be seen by the camera associated angle is
%       equal to -1
%

% Get camera field of vision
% [pcam,lcam]=camera(hCam);
% betaCam = 21 ;
% etaCam = 27 ;
% [pcam, lcam] = cameraAnalytic(hCam,90-alphaCam, betaCam, etaCam);

% Convert Obstacles positions to robot reference
[vx,vy] = world2robot(robotPos(1),robotPos(2),robotTheta,ObstaclesVertices(:,1),ObstaclesVertices(:,2));

[~, ~, ~, ~, ua, ub] = lineSegmentsIntersection(0, 0,...
    cosd(single(armAngle)), sind(single(armAngle)), vx(ObstaclesEdges(:,1)),...
    vy(ObstaclesEdges(:,1)), vx(ObstaclesEdges(:,2)), vy(ObstaclesEdges(:,2)));

isOnRange = (ua >= 10) & (ua <= 80) & (ub >= 0) & (ub <= 1);

if nnz(isOnRange)==0
    armDist = int8(-1);
else
    armDist = int8(min(ua(isOnRange)));
end


end

function [x_new,y_new]=world2robot(x_robot,y_robot,theta_robot,x_world,y_world)
% WORLD2ROBOT Convert coordinates from world to robot
%
% Inputs
%   - x_robot: Robot X position (in world reference)
%   - y_robot: Robot Y position (in world reference)
%   - theta_robot: Robot angle  (in world reference)
%   - x_world: X value(s) to convert (in world reference)
%   - y_world: Y value(s) to convert (in world reference)
%
% Outpus
%   - x_new: Point(s) coordinate (X) in robot reference
%   - y_new: Point(s) coordinate (Y) in robot reference

% Translate coordinates reference
x_dif=x_world-x_robot;
y_dif=y_world-y_robot;

% Rotate coordinates reference
% x_new=x_dif*cosd(theta_robot)-y_dif*sind(theta_robot);
% y_new=x_dif*sind(theta_robot)+y_dif*cosd(theta_robot);
x_new = cosd(theta_robot)*x_dif + sind(theta_robot)*y_dif;
y_new = cosd(theta_robot)*y_dif - sind(theta_robot)*x_dif;
% see http://www.mathematics-online.org/inhalt/aussage/aussage444/

% TODO We have identified that the sign of converted coordinates is the
% opposite of the expected but we don't have an explanation for that
% x_new = -x_new;
% y_new = -y_new;

end

== stateflow chart variant_2_MRC_SimulationModel/RobotModel/Sensors Camera_Distance/Distance_sensor/Scanner ==
  state ScanDistance
    state Scanning
      state LookFront
        entry:
        ArmAngle = int8(0);
        exit:
        scanner_value(DistanceSensorPosition.MIDDLE) = ArmDist;
        scanner_status = DistanceSensorPosition.MIDDLE;
      state LookLeft
        entry:
        ArmAngle = int8(25);
        exit:
        scanner_value(DistanceSensorPosition.LEFT) = ArmDist;
        scanner_status = DistanceSensorPosition.LEFT;
      state LookRight
        entry:
        ArmAngle = int8(-25);
        exit:
        scanner_value(DistanceSensorPosition.RIGHT) = ArmDist;
        scanner_status = DistanceSensorPosition.RIGHT;
      (default) -> LookFront : {
          | scanner_value = int8(-1*ones(1,3));
          | scanner_status = DistanceSensorPosition.NO;
          | }
      LookLeft -> LookFront [order 1] : after(4,tick)
      LookLeft -> LookFront [order 2] : [after(3,tick) && ArmDist == -1]
      LookFront -> LookRight [order 1] : after(3,tick)
      LookFront -> LookRight [order 2] : [after(2,tick) && ArmDist == -1]
      LookRight -> LookLeft [order 1] : after(3,tick)
      LookRight -> LookLeft [order 2] : [after(2,tick) && ArmDist == -1]
    state Idle
      entry:
      ArmAngle = int8(0);
      during,exit:
      scanner_value = int8(-1*ones(1,3));
      scanner_status = DistanceSensorPosition.NO;
    (default) -> Scanning
    Scanning -> Idle : pauseScanner
    Idle -> Scanning : resumeScanner
  data: ArmDist input; scanner_status output Enum: DistanceSensorPosition; scanner_value output int8; ArmAngle output
  events: resumeScanner local FUNCTION_CALL_EVENT; pauseScanner local FUNCTION_CALL_EVENT

== stateflow chart variant_2_MRC_SimulationModel/InputProcessing/Estimator ==
  settings: sampleTime=Ts
  state Navigation [parallel]
    settings: executionOrder=2
    state Normal
      entry,during:
      if abs(correction) >= single(99)
      DistanceRemainToTarget = single(0);
      BearingRemainToTarget = single(5);
      else
      DistanceRemainToTarget = single(30) ;
      BearingRemainToTarget = single(0+correction);
      end
    state GoToTarget
      state TargetInView
        entry,during:
        [~,ind] = min(DistanceCameraTargets(DistanceCameraTargets>0));
        DistanceToTarget=single(DistanceCameraTargets(ind));
        DistanceRemainToTarget=DistanceToTarget;
        BearingToTarget= single(BearingCameraTargets(ind))/2;
        BearingRemainToTarget=BearingToTarget + correction;
        ResetEncoder;
      state TargetHidden
        entry,during:
        DistanceRemainToTarget=DistanceToTarget-CurrentDistance;
        BearingRemainToTarget=BearingToTarget-CurrentBearing;
      (default) -> TargetInView
      TargetInView -> TargetHidden [order 1] : [DistanceRemainToTarget<35]
    state SearchTargetAround
      state GoBackToZero
        entry:
        DistanceRemainToTarget=single(0);
        BearingRemainToTarget=single(-10);
        ResetEncoder;
      state SearchLeftTarget
        entry:
        DistanceRemainToTarget=single(0);
        BearingRemainToTarget=single(-5);
        ResetEncoder;
      state SearchRightTarget
        entry:
        DistanceRemainToTarget=single(0);
        BearingRemainToTarget=single(5);
        ResetEncoder;
      (default) -> SearchLeftTarget
      SearchRightTarget -> GoBackToZero : [CurrentBearing >= 180]
      SearchLeftTarget -> SearchRightTarget : [CurrentBearing <= -90]
    state Wait_for_scoring
      entry:
      DistanceRemainToTarget = single(0);
      BearingRemainToTarget = single(0);
      ResetEncoder;
    (default) -> Normal
    Normal -> GoToTarget : [DistanceCameraTargets(1) ~= 0]
    TargetInView -> Normal [order 2] : [DistanceCameraTargets(1) == 0]
    GoBackToZero -> Normal : [CurrentBearing <= -90]
    SearchTargetAround -> GoToTarget : [DistanceCameraTargets(1) ~= 0]
    GoToTarget -> Wait_for_scoring : [ DistanceRemainToTarget < 15]
    Wait_for_scoring -> SearchTargetAround : after(3,sec)
  state ObstacleAvoidance [parallel]
    settings: executionOrder=1
    state NoCorrection
      entry:
      correction = single(0);
    state AvoidRight
      entry:
      correction = single(10);
    state AvoidLeft
      entry:
      correction = single(-10);
    state AvoidMiddle
      entry:
      correction = bsign * single(99);
    (default) -> NoCorrection
    NoCorrection -> AvoidRight [order 2] : [scanner_status == DistanceSensorPosition.RIGHT && ...
        | scanner_values(DistanceSensorPosition.RIGHT) > -1]
    NoCorrection -> AvoidLeft [order 1] : [scanner_status == DistanceSensorPosition.LEFT && ...
        | scanner_values(DistanceSensorPosition.LEFT) > -1]
    AvoidRight -> NoCorrection [order 1] : [scanner_status == DistanceSensorPosition.RIGHT && ...
        | scanner_values(DistanceSensorPosition.RIGHT) == -1]
    AvoidLeft -> NoCorrection [order 1] : [scanner_status == DistanceSensorPosition.LEFT && ...
        | scanner_values(DistanceSensorPosition.LEFT) == -1]
    AvoidRight -> NoCorrection [order 2] : [scanner_status == DistanceSensorPosition.LEFT && ...
        | scanner_values(DistanceSensorPosition.LEFT) > -1]
    AvoidRight -> AvoidMiddle [order 3] : [scanner_status == DistanceSensorPosition.MIDDLE && ...
        | scanner_values(DistanceSensorPosition.MIDDLE) > -1]
        | {bsign = single(1);}
    AvoidLeft -> NoCorrection [order 2] : [scanner_status == DistanceSensorPosition.RIGHT && ...
        | scanner_values(DistanceSensorPosition.RIGHT) > -1]
    NoCorrection -> AvoidMiddle [order 3] : [scanner_status == DistanceSensorPosition.MIDDLE && ...
        | scanner_values(DistanceSensorPosition.MIDDLE) > -1]
        | {bsign = single(sign(rand-0.5));}
    AvoidMiddle -> NoCorrection : [scanner_status == DistanceSensorPosition.MIDDLE && ...
        | scanner_values(DistanceSensorPosition.MIDDLE) == -1]
    AvoidLeft -> AvoidMiddle [order 3] : [scanner_status == DistanceSensorPosition.MIDDLE && ...
        | scanner_values(DistanceSensorPosition.MIDDLE) > -1]
        | {bsign = single(-1);}
  data: bsign local single; BearingRemainToTarget output single size=1; DistanceRemainToTarget output single size=1; DistanceCameraTargets input int16; BearingCameraTargets input int8; scanner_status input Enum: DistanceSensorPosition; scanner_values input size=[1 3]; CurrentDistance input single; CurrentBearing input single; BearingToTarget local single; DistanceToTarget local single; ind local; correction local single
  events: ResetEncoder output EITHER_EDGE_EVENT

== stateflow chart variant_2_MRC_SimulationModel/Scoring/Referee/Referee ==
  state Standby
    entry:
    numTargets = size(SitesPositions,1);
    targetsFound = false(size(SitesPositions,1),1);
    timeLastTargetFound = 0;
    elapsedTime = 0;
    numTargetsFound = 0;
    allowedRunTime = 180;
    startingRadius = 10;
    targetBoundaryRadius = 7;
    statTimeReq = 2.5;
  state Running
    entry: startTiming;
    during:
    elapsedTime = getTiming;
    [nearLocation, currentTarget] = testIfNearLocation(robotPosition, SitesPositions, targetBoundaryRadius);
    state NearLocation
      entry: snapshotTime = elapsedTime;
    state Roaming
    Roaming -> NearLocation : [nearLocation == true]
    (default) -> Roaming
    NearLocation -> Roaming [order 2] : [nearLocation == false]
    NearLocation -> (junction 43) [order 1] : [(elapsedTime - snapshotTime) > statTimeReq]
    (junction 44) -> Roaming
    (junction 43) -> (junction 44) : {[targetsFound, timeLastTargetFound] = ...
        | updateTargetsFound(targetsFound, currentTarget, timeLastTargetFound,elapsedTime);
        | numTargetsFound = sum(targetsFound);}
  state Finished
  (default) -> Standby
  Finished -> Standby : [StartFlag == false]
  Standby -> Running : [StartFlag == true &&...
      | distancefrom(robotPosition, startPos) < startingRadius ]
  Running -> Standby [order 2] : [StartFlag == false]
  Running -> Finished [order 1] : [numTargetsFound == numTargets ||...
      |  elapsedTime >= allowedRunTime-sqrt(eps)]
  data: et function_output; tfound_in function_input; currentT function_input; tfound_out function_output; lastTime_in function_input; lastTime_out function_output; time function_input; robotPos function_input; targetPos function_input; proximityVal function_input; nearLoc function_output; currentLoc function_output; pos function_input; x0 function_input; d function_output; startPos parameter; allowedRunTime local; statTimeReq local; startingRadius local; robotPosition input; targetBoundaryRadius local; StartFlag input; SitesPositions parameter; timeLastTargetFound output; nearLocation local; numTargetsFound local; elapsedTime output; numTargets local; currentTarget local; targetsFound output; snapshotTime local; local_t local; sim_time input
  function startTiming:
    | function startTiming
    | global local_t sim_time
    | 
    | if strcmp(coder.target,'rtw')
    |     coder.ceval('tic',int32(2));
    | else
    |     local_t = sim_time;
    | end
  function et = getTiming:
    | function et = getTiming
    | global sim_time local_t
    | 
    | lt = 0;
    | 
    | if strcmp(coder.target,'rtw')
    |     coder.ceval('toc',coder.wref(lt),int32(2));
    | else
    |     lt = sim_time - local_t;
    | end
    | 
    | et = lt;
  function [tfound_out, lastTime_out] = updateTargetsFound(tfound_in, currentT, lastTime_in, time):
    | function [tfound_out, lastTime_out] = updateTargetsFound(tfound_in, currentT, lastTime_in, time)
    | 
    | if any(tfound_in & currentT) %is this an existing target
    |     lastTime_out = lastTime_in;
    | else
    |     lastTime_out = time;
    | end
    | 
    | tfound_out = tfound_in | currentT; %update list of found targets
  function [nearLoc, currentLoc] = testIfNearLocation(robotPos, targetPos, proximityVal):
    | function [nearLoc, currentLoc] = testIfNearLocation(robotPos, targetPos, proximityVal)
    | %#codegen
    | delta = bsxfun(@minus, targetPos, robotPos);
    | dist = sum(delta.^2,2);
    | 
    | currentLoc = dist <= proximityVal^2;
    | nearLoc = any(currentLoc);
  function d = distancefrom(pos,x0):
    | function d = distancefrom(pos,x0)
    | d = sqrt(sum((pos-x0).^2));

== matlab function variant_2_MRC_SimulationModel/Scoring/FigureOutput/call_plotFigure ==
  data: X input; SitesPositions parameter; T_found input; t_last input; t input; T_located input; pcam parameter; lcam parameter; robotheta input; ArmAngleEstimated input; ArmAngleCommand input; DisplayPositions input
function fcn(X, SitesPositions, T_found, t_last, t, T_located,pcam,lcam,robotheta,...
    ArmAngleEstimated, ArmAngleCommand, DisplayPositions)
coder.extrinsic('plotFigure');

plotFigure(X, SitesPositions, T_found, t_last, t, T_located,pcam,lcam,robotheta,...
    single(ArmAngleEstimated), single(ArmAngleCommand), DisplayPositions);
